simulink model "problem3"  (R2020b)
settings: Solver=FixedStepAuto  StartTime=0.0  StopTime=10.0  FixedStep=0.01  RelTol=1e-3
PostLoadFcn:
  | m=1000;
  | b=50;
  | r=10;
  | Kp=93563.6529;
  | Ki=3004.6442;
  | u=5;
settings Model: Creator=sansh  LastModifiedBy=Gopinath Murugan
settings DataIOCC: ReturnWorkspaceOutputs=off
settings DebuggingCC: ArithmeticOperatorsInVariantConditions=warning
settings SFSimCC: SimUseLocalCustomCode=off  CustomCodeUndefinedFunction=UseInterfaceOnly
settings RTWCC: RTWUseLocalCustomCode=off
settings CodeAppCC: StateflowObjectComments=on

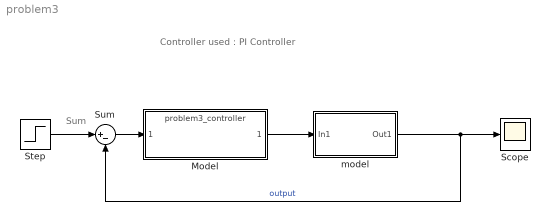
== system problem3 ==
  note: Controller used : PI Controller
  note: Sum
  Model : ModelReference  ModelNameDialog=problem3_controller.slx  SimulationMode=Normal  ModelReferenceVersion=1.2
  Scope : Scope
  Step : Step  Time=0  After=u  SampleTime=0
  Sum : Sum  Inputs=|+-
  model : Subsystem
  wires:
  model/1(Out1) -> Sum/2, Scope/1  "output"
  Step/1 -> Sum/1
  Sum/1 -> Model/1
  Model/1 -> model/1(In1)

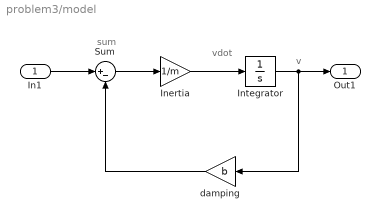
== system problem3/model ==
  note: vdot
  note: sum
  note: v
  In1 : Inport
  Inertia : Gain  Gain=1/m
  Integrator : Integrator
  Sum : Sum  Inputs=|+-
  damping : Gain  Gain=b
  Out1 : Outport
  wires:
  In1/1 -> Sum/1
  Sum/1 -> Inertia/1
  Inertia/1 -> Integrator/1
  damping/1 -> Sum/2
  Integrator/1 -> Out1/1, damping/1
